simulink model "qam"  (R2019a)
settings: Solver=VariableStepAuto  StartTime=0.0  StopTime=10.0  RelTol=1e-3
libraries: visionsources x1
settings Model: Creator=DSP_08  LastModifiedBy=harsh
settings DataIOCC: ReturnWorkspaceOutputs=off
settings DebuggingCC: ArithmeticOperatorsInVariantConditions=warning

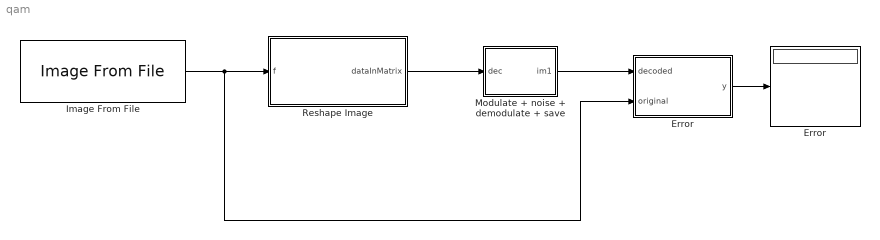
== system qam ==
  Error : MATLAB Function  TreatAsAtomicUnit=on
  "Error " : Display
  Image From File : visionsources/Image From File  Tag=vipblks_nd  FileName=E:\LNMIIT_Study\Sem 6\Lab\Design Lab\Project1\Matlab\rec.bmp  Ts=inf  imagePorts=One multidimensional signal  OutPortLabels=R|G|B  ImageDataType=Inherit from input image  sdImageDataType=uint(8)  Signed=on  WordLength=16  FractionLengthMode=User-defined  FractionLength=15
      settings: SourceProductName=Computer Vision Toolbox
  "Modulate + noise + demodulate + save " : MATLAB Function  TreatAsAtomicUnit=on
  "Reshape Image " : MATLAB Function  TreatAsAtomicUnit=on
  wires:
  Image From File/1 -> Error/2(original), "Reshape Image "/1(f)
  "Reshape Image "/1(dataInMatrix) -> "Modulate + noise + demodulate + save "/1(dec)
  "Modulate + noise + demodulate + save "/1(im1) -> Error/1(decoded)
  Error/1(y) -> "Error "/1

== matlab function qam/Modulate + noise + demodulate + save  ==
  data: dec input; im1 output
function im1 = fcn(dec)
n = length(dec);
out = zeros(n,1) + 1j*zeros(n,1);
for i =1:n
    a = 0+ 1j*0;
    if(bi2de(dec(i,1:3),'left-msb')==0)
        a=a+ -7;
    elseif(bi2de(dec(i,1:3),'left-msb')==1)
             a=a+ -5;
    elseif(bi2de(dec(i,1:3),'left-msb')==3)
             a=a+ -3;
    elseif(bi2de(dec(i,1:3),'left-msb')==2)
             a=a+ -1;
    elseif(bi2de(dec(i,1:3),'left-msb')==6)
             a=a+ 1;
    elseif(bi2de(dec(i,1:3),'left-msb')==4)
             a=a+ 3;
    elseif(bi2de(dec(i,1:3),'left-msb')==5)
             a=a+ 5;
    elseif(bi2de(dec(i,1:3),'left-msb')==7)
             a=a+ 7;   
                    
    end
    
    
    if(bi2de(dec(i,4:6),'left-msb')==0)
        a=a+ -1j*7;
    elseif(bi2de(dec(i,4:6),'left-msb')==1)
             a=a+ -1j*5;
    elseif(bi2de(dec(i,4:6),'left-msb')==3)
             a=a+ -1j*3;
    elseif(bi2de(dec(i,4:6),'left-msb')==2)
             a=a+ -1j*1;
    elseif(bi2de(dec(i,4:6),'left-msb')==6)
             a=a+ 1j*1;
    elseif(bi2de(dec(i,4:6),'left-msb')==4)
             a=a+ 1j*3;
    elseif(bi2de(dec(i,4:6),'left-msb')==5)
             a=a+ 1j*5;
    elseif(bi2de(dec(i,4:6),'left-msb')==7)
             a=a+ 1j*7; 
    end
    out(i) = a;
end

snr_db = 0:2:24;
snr_lin = 10.^(snr_db/10);
N0 = 1./(snr_lin);
N=length(out);
gnoise = randn(N,1) + 1j*randn(N,1);
out = out+gnoise*sqrt(N0(8));
sig = round(out);

n = length(sig);
out1 = zeros(n,6);
a = zeros(1,6);

for i =1:n
    
    switch real(sig(i))
        case -7
            a(1:3)=[0 0 0];
        case -5
            a(1:3)=[0 0 1];
        case -3
            a(1:3)=[0 1 1];
        case -1
            a(1:3)=[0 1 0];
        case 1
            a(1:3)=[1 1 0];
        case 3
            a(1:3)=[1 0 0];
        case 5
            a(1:3)=[1 0 1];
        case 7
            a(1:3)=[1 1 1];
        
    end
    switch imag(sig(i))
        case -7
            a(4:6)=[0 0 0];
        case -5
            a(4:6)=[0 0 1];
        case -3
            a(4:6)=[0 1 1];
        case -1
            a(4:6)=[0 1 0];
        case 1
            a(4:6)=[1 1 0];
        case 3
            a(4:6)=[1 0 0];
        case 5
            a(4:6)=[1 0 1];
        case 7
            a(4:6)=[1 1 1];
        
    end
    
    out1(i,:) = a;
end

coder.extrinsic('imwrite');
dataOut1 = logical(out1(:));
dataOut1 = dataOut1(1:length(dataOut1)-rem(uint64(length(dataOut1)),uint64(sqrt(length(dataOut1)))));
im1 = reshape(dataOut1,[],uint64(sqrt(length(dataOut1))));
imwrite(im1,'sim.bmp');

end

== matlab function qam/Reshape Image  ==
  data: f input; dataInMatrix output
function dataInMatrix = fcn(f)
b = f(:)';
if rem(length(b),6)~=0
    b1 = [b zeros(1,6-rem(length(b),6))];
end
dataInMatrix = reshape(b1,[],6);
end

== matlab function qam/Error ==
  data: decoded input; y output; original input
function y = fcn(decoded,original)
coder.extrinsic("mse");
y = zeros(1,1);
y = mse(decoded(:),original(:));
end
